simulink model "ServoControl2D"  (R2015b)
settings: Solver=VariableStepAuto  StartTime=0.0  StopTime=10.0  RelTol=1e-3
values from neighbouring files (symbols this model uses):
  De = 7.7*10^(-6)    (= 7.7e-06)    [Servo_Control2D.m]
  Je = 5.3*10^(-7)    (= 5.3e-07)    [Servo_Control2D.m]
  Kp = 0.3    [Servo_Control2D.m]
  Kt = 7.67*10^(-3)    (= 0.00767)    [Servo_Control2D.m]
  La = 180*10^(-6)    (= 0.00018)    [Servo_Control2D.m]
  Ra = 2.6    [Servo_Control2D.m]
  Td = Ti/4    (= 0.05)    [Servo_Control2D.m]
  Ti = 0.2    [Servo_Control2D.m]
settings Model: Creator=kenny  LastModifiedBy=kenny

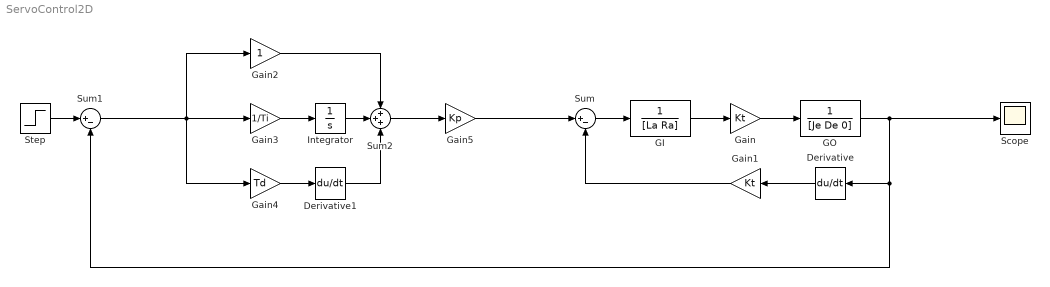
== system ServoControl2D ==
  Derivative : Derivative
  Derivative1 : Derivative
  GI : TransferFcn  Denominator=[La Ra]
  GO : TransferFcn  Denominator=[Je De 0]
  Gain : Gain  Gain=Kt
  Gain1 : Gain  Gain=Kt
  Gain2 : Gain
  Gain3 : Gain  Gain=1/Ti
  Gain4 : Gain  Gain=Td
  Gain5 : Gain  Gain=Kp
  Integrator : Integrator
  Scope : Scope
  Step : Step  SampleTime=0
  Sum : Sum  Inputs=|+-
  Sum1 : Sum  Inputs=|+-
  Sum2 : Sum  Inputs=+++
  wires:
  GI/1 -> Gain/1
  Gain/1 -> GO/1
  Derivative/1 -> Gain1/1
  Gain1/1 -> Sum/2
  Sum/1 -> GI/1
  Step/1 -> Sum1/1
  GO/1 -> Sum1/2, Derivative/1, Scope/1
  Gain4/1 -> Derivative1/1
  Gain3/1 -> Integrator/1
  Integrator/1 -> Sum2/2
  Derivative1/1 -> Sum2/3
  Gain2/1 -> Sum2/1
  Sum2/1 -> Gain5/1
  Sum1/1 -> Gain4/1, Gain2/1, Gain3/1
  Gain5/1 -> Sum/1
